simulink model "amon_model_full"  (R2025b)
settings: Solver=VariableStepAuto  StartTime=0.0  StopTime=1  RelTol=1e-3
values from neighbouring files (symbols this model uses):
  EDF_max = 100    [amon_model.m]
  EDF_min = 0    [amon_model.m]
  f_0_T = [0; 0; 0]    [amon_model.m]
  g = [0; 0; 9.81]    [amon_model.m]
  J = [0.02 0 0; 0 0.018 0; 0 0 0.03]    [amon_model.m]
  K_d = 0    [amon_model.m]
  k_fins = [1 1 1 1]    [amon_model.m]
  m = 2253    [amon_model.m]
  n_fins = [0  0  1 -1 ... (first row only)    [amon_model.m]
  r_fins = [   0.50  -0.50      0      0 ... (first row only)    [amon_model.m]
  r_T = [0; 0; 0]    [amon_model.m]
  servo1_offset = 0    [amon_model.m]
  servo2_offset = 0    [amon_model.m]
  servo3_offset = 0    [amon_model.m]
  servo4_offset = 0    [amon_model.m]
  servo_max = -45    [amon_model.m]
  servo_min = -45    [amon_model.m]
  tau_0_T = [0; 0; 0]    [amon_model.m]
  tau_edf = 0.2    [amon_model.m]
  tau_servo = 0.2    [amon_model.m]
libraries: aerolibconvert2 x4
settings Model: Creator=titit  LastModifiedBy=titit

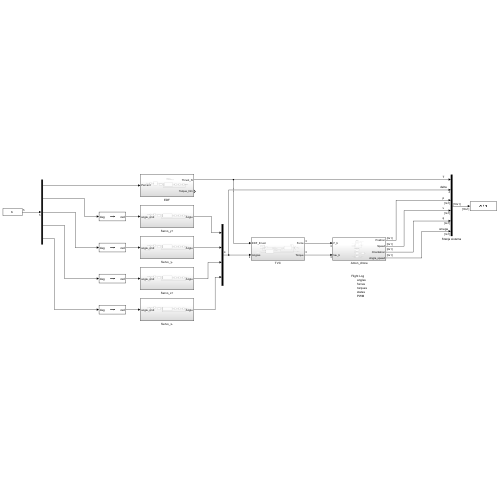
[thumbnail: Simulink's stored preview of the top-level diagram]
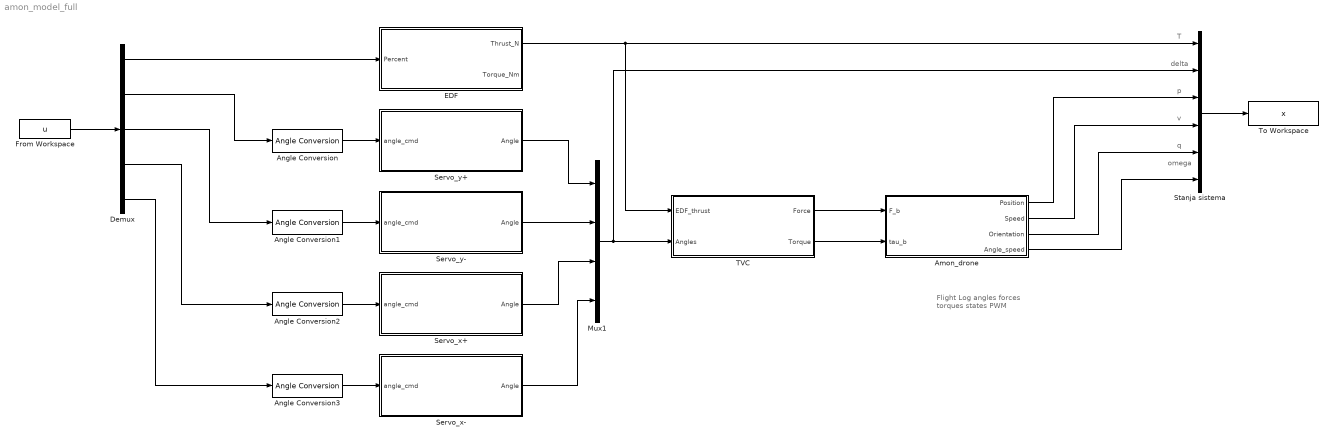
== system amon_model_full ==
  note: Flight Log
      | 	angles
      | 	forces
      | 	torques
      | 	states
      | 	PWM
  note: T
  note: delta
  note: p
  note: v
  note: q
  note: omega
  Amon_drone : Subsystem
  Angle Conversion{,1..3} (4 alike) : aerolibconvert2/Angle Conversion  IU=deg  OU=rad
  Demux : Demux  Outputs=5
  EDF : Subsystem
  From Workspace : FromWorkspace  VariableName=u
  Mux1 : Mux
  Servo_x+ : Subsystem
  Servo_x- : Subsystem
  Servo_y+ : Subsystem
  Servo_y- : Subsystem
  Stanja sistema : Mux  Inputs=6
  TVC : Subsystem
  To Workspace : ToWorkspace  VariableName=x  SaveFormat=Timeseries  SampleTime=-1
  wires:
  From Workspace/1 -> Demux/1
  Stanja sistema/1 -> To Workspace/1
  Demux/1 -> EDF/1(Percent)
  Demux/2 -> Angle Conversion/1
  Demux/3 -> Angle Conversion1/1
  Demux/4 -> Angle Conversion2/1
  Demux/5 -> Angle Conversion3/1
  Angle Conversion/1 -> Servo_y+/1(angle_cmd)
  Angle Conversion1/1 -> Servo_y-/1(angle_cmd)
  Angle Conversion2/1 -> Servo_x+/1(angle_cmd)
  Angle Conversion3/1 -> Servo_x-/1(angle_cmd)
  Servo_y+/1(Angle) -> Mux1/1
  Servo_y-/1(Angle) -> Mux1/2
  Servo_x+/1(Angle) -> Mux1/3
  Servo_x-/1(Angle) -> Mux1/4
  Mux1/1 -> Stanja sistema/2, TVC/2(Angles)
  EDF/1(Thrust_N) -> TVC/1(EDF_thrust), Stanja sistema/1
  TVC/1(Force) -> Amon_drone/1(F_b)
  TVC/2(Torque) -> Amon_drone/2(tau_b)
  Amon_drone/1(Position) -> Stanja sistema/3
  Amon_drone/2(Speed) -> Stanja sistema/4
  Amon_drone/3(Orientation) -> Stanja sistema/5
  Amon_drone/4(Angle_speed) -> Stanja sistema/6

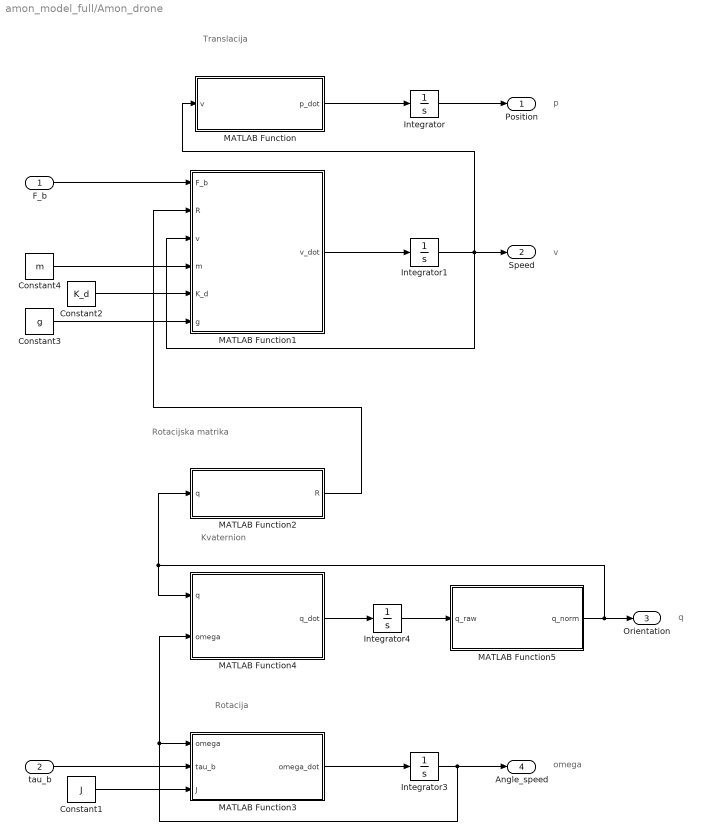
== system amon_model_full/Amon_drone ==
  note: p
  note: v
  note: q
  note: omega
  note: Translacija
  note: Kvaternion
  note: Rotacijska matrika
  note: Rotacija
  F_b : Inport
  tau_b : Inport  Port=2
  Constant1 : Constant  Value=J
  Constant2 : Constant  Value=K_d
  Constant3 : Constant  Value=g
  Constant4 : Constant  Value=m
  Integrator : Integrator
  Integrator1 : Integrator
  Integrator3 : Integrator  InitialCondition=[0;0;0]
  Integrator4 : Integrator
  MATLAB Function : MATLAB Function  TreatAsAtomicUnit=on
  MATLAB Function1 : MATLAB Function  TreatAsAtomicUnit=on
  MATLAB Function2 : MATLAB Function  TreatAsAtomicUnit=on
  MATLAB Function3 : MATLAB Function  TreatAsAtomicUnit=on
  MATLAB Function4 : MATLAB Function  TreatAsAtomicUnit=on
  MATLAB Function5 : MATLAB Function  TreatAsAtomicUnit=on
  Position : Outport
  Speed : Outport  Port=2
  Orientation : Outport  Port=3
  Angle_speed : Outport  Port=4
  wires:
  MATLAB Function/1(p_dot) -> Integrator/1
  Integrator/1 -> Position/1
  Integrator1/1 -> MATLAB Function/1(v), MATLAB Function1/3(v), Speed/1
  MATLAB Function1/1(v_dot) -> Integrator1/1
  MATLAB Function3/1(omega_dot) -> Integrator3/1
  Integrator3/1 -> MATLAB Function3/1(omega), MATLAB Function4/2(omega), Angle_speed/1
  F_b/1 -> MATLAB Function1/1(F_b)
  Constant4/1 -> MATLAB Function1/4(m)
  Constant2/1 -> MATLAB Function1/5(K_d)
  Constant3/1 -> MATLAB Function1/6(g)
  MATLAB Function2/1(R) -> MATLAB Function1/2(R)
  Constant1/1 -> MATLAB Function3/3(J)
  tau_b/1 -> MATLAB Function3/2(tau_b)
  MATLAB Function4/1(q_dot) -> Integrator4/1
  Integrator4/1 -> MATLAB Function5/1(q_raw)
  MATLAB Function5/1(q_norm) -> Orientation/1, MATLAB Function2/1(q), MATLAB Function4/1(q)

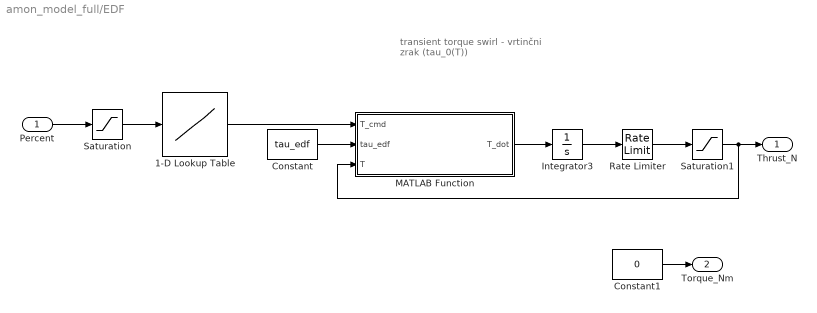
== system amon_model_full/EDF ==
  note: transient torque
      | swirl - vrtinčni zrak (tau_0(T))
  Percent : Inport
  1-D Lookup Table : Lookup_n-D  NumberOfTableDimensions=1  BreakpointsForDimension1=[-5:5]  Table=tanh([-5:5])  InternalRulePriority=Speed  RndMeth=Simplest
  Constant : Constant  Value=tau_edf
  Constant1 : Constant  Value=0
  Integrator3 : Integrator
  MATLAB Function : MATLAB Function  TreatAsAtomicUnit=on
  Rate Limiter : RateLimiter  SampleTimeMode=inherited
  Saturation : Saturate  UpperLimit=EDF_max  LowerLimit=EDF_min
  Saturation1 : Saturate  UpperLimit=100  LowerLimit=0
  Thrust_N : Outport
  Torque_Nm : Outport  Port=2
  wires:
  Percent/1 -> Saturation/1
  1-D Lookup Table/1 -> MATLAB Function/1(T_cmd)
  MATLAB Function/1(T_dot) -> Integrator3/1
  Saturation/1 -> 1-D Lookup Table/1
  Constant/1 -> MATLAB Function/2(tau_edf)
  Rate Limiter/1 -> Saturation1/1
  Saturation1/1 -> MATLAB Function/3(T), Thrust_N/1
  Constant1/1 -> Torque_Nm/1
  Integrator3/1 -> Rate Limiter/1

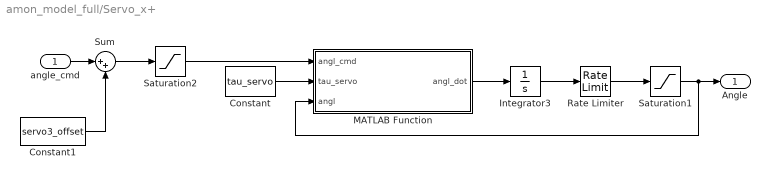
== system amon_model_full/Servo_x+ ==
  angle_cmd : Inport
  Constant : Constant  Value=tau_servo
  Constant1 : Constant  Value=servo3_offset
  Integrator3 : Integrator
  MATLAB Function : MATLAB Function  TreatAsAtomicUnit=on
  Rate Limiter : RateLimiter  SampleTimeMode=inherited
  Saturation1 : Saturate  UpperLimit=servo_max  LowerLimit=servo_min
  Saturation2 : Saturate  UpperLimit=servo_max  LowerLimit=servo_min
  Sum : Sum  Inputs=|++
  Angle : Outport
  wires:
  Sum/1 -> Saturation2/1
  Constant/1 -> MATLAB Function/2(tau_servo)
  MATLAB Function/1(angl_dot) -> Integrator3/1
  Saturation2/1 -> MATLAB Function/1(angl_cmd)
  Constant1/1 -> Sum/2
  angle_cmd/1 -> Sum/1
  Saturation1/1 -> MATLAB Function/3(angl), Angle/1
  Rate Limiter/1 -> Saturation1/1
  Integrator3/1 -> Rate Limiter/1

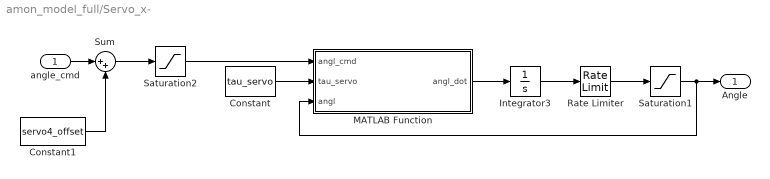
== system amon_model_full/Servo_x- ==
  angle_cmd : Inport
  Constant : Constant  Value=tau_servo
  Constant1 : Constant  Value=servo4_offset
  Integrator3 : Integrator
  MATLAB Function : MATLAB Function  TreatAsAtomicUnit=on
  Rate Limiter : RateLimiter  SampleTimeMode=inherited
  Saturation1 : Saturate  UpperLimit=servo_max  LowerLimit=servo_min
  Saturation2 : Saturate  UpperLimit=servo_max  LowerLimit=servo_min
  Sum : Sum  Inputs=|++
  Angle : Outport
  wires:
  Constant/1 -> MATLAB Function/2(tau_servo)
  MATLAB Function/1(angl_dot) -> Integrator3/1
  Saturation2/1 -> MATLAB Function/1(angl_cmd)
  Constant1/1 -> Sum/2
  angle_cmd/1 -> Sum/1
  Saturation1/1 -> MATLAB Function/3(angl), Angle/1
  Rate Limiter/1 -> Saturation1/1
  Sum/1 -> Saturation2/1
  Integrator3/1 -> Rate Limiter/1

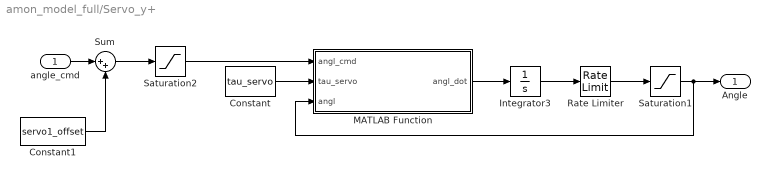
== system amon_model_full/Servo_y+ ==
  angle_cmd : Inport
  Constant : Constant  Value=tau_servo
  Constant1 : Constant  Value=servo1_offset
  Integrator3 : Integrator
  MATLAB Function : MATLAB Function  TreatAsAtomicUnit=on
  Rate Limiter : RateLimiter  SampleTimeMode=inherited
  Saturation1 : Saturate  UpperLimit=servo_max  LowerLimit=servo_min
  Saturation2 : Saturate  UpperLimit=servo_max  LowerLimit=servo_min
  Sum : Sum  Inputs=|++
  Angle : Outport
  wires:
  Saturation2/1 -> MATLAB Function/1(angl_cmd)
  MATLAB Function/1(angl_dot) -> Integrator3/1
  Saturation1/1 -> MATLAB Function/3(angl), Angle/1
  Constant/1 -> MATLAB Function/2(tau_servo)
  Rate Limiter/1 -> Saturation1/1
  angle_cmd/1 -> Sum/1
  Sum/1 -> Saturation2/1
  Constant1/1 -> Sum/2
  Integrator3/1 -> Rate Limiter/1

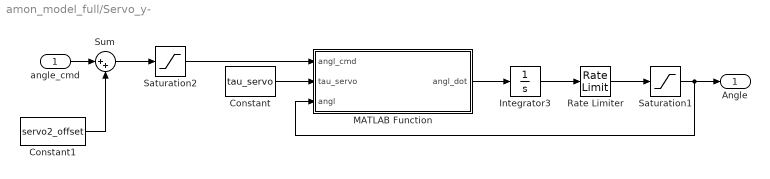
== system amon_model_full/Servo_y- ==
  angle_cmd : Inport
  Constant : Constant  Value=tau_servo
  Constant1 : Constant  Value=servo2_offset
  Integrator3 : Integrator
  MATLAB Function : MATLAB Function  TreatAsAtomicUnit=on
  Rate Limiter : RateLimiter  SampleTimeMode=inherited
  Saturation1 : Saturate  UpperLimit=servo_max  LowerLimit=servo_min
  Saturation2 : Saturate  UpperLimit=servo_max  LowerLimit=servo_min
  Sum : Sum  Inputs=|++
  Angle : Outport
  wires:
  Sum/1 -> Saturation2/1
  Constant/1 -> MATLAB Function/2(tau_servo)
  MATLAB Function/1(angl_dot) -> Integrator3/1
  Saturation2/1 -> MATLAB Function/1(angl_cmd)
  Constant1/1 -> Sum/2
  angle_cmd/1 -> Sum/1
  Saturation1/1 -> MATLAB Function/3(angl), Angle/1
  Rate Limiter/1 -> Saturation1/1
  Integrator3/1 -> Rate Limiter/1

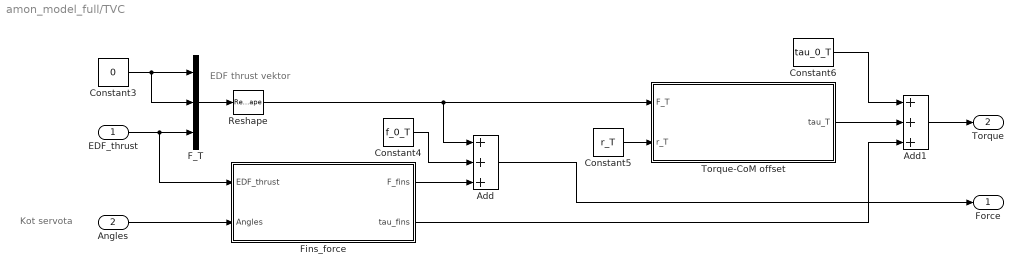
== system amon_model_full/TVC ==
  note: EDF thrust vektor
  note: Kot servota
  EDF_thrust : Inport
  Angles : Inport  Port=2
  Add : Sum  Inputs=+++
  Add1 : Sum  Inputs=+++
  Constant3 : Constant  Value=0
  Constant4 : Constant  Value=f_0_T
  Constant5 : Constant  Value=r_T
  Constant6 : Constant  Value=tau_0_T
  F_T : Mux  Inputs=3
  Fins_force : Subsystem
  Reshape : Reshape  OutputDimensionality=Column vector (2-D)
  Torque-CoM offset : Subsystem
  Force : Outport
  Torque : Outport  Port=2
  wires:
  EDF_thrust/1 -> Fins_force/1(EDF_thrust), F_T/3
  Constant3/1 -> F_T/2, F_T/1
  Angles/1 -> Fins_force/2(Angles)
  F_T/1 -> Reshape/1
  Constant5/1 -> Torque-CoM offset/2(r_T)
  Constant6/1 -> Add1/1
  Torque-CoM offset/1(tau_T) -> Add1/2
  Fins_force/2(tau_fins) -> Add1/3
  Add1/1 -> Torque/1
  Add/1 -> Force/1
  Fins_force/1(F_fins) -> Add/3
  Constant4/1 -> Add/2
  Reshape/1 -> Torque-CoM offset/1(F_T), Add/1

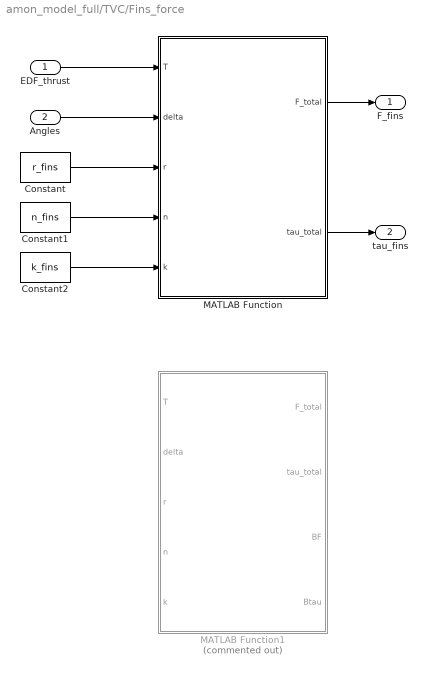
== system amon_model_full/TVC/Fins_force ==
  EDF_thrust : Inport
  Angles : Inport  Port=2
  Constant : Constant  Value=r_fins
  Constant1 : Constant  Value=n_fins
  Constant2 : Constant  Value=k_fins
  MATLAB Function : MATLAB Function  TreatAsAtomicUnit=on
  MATLAB Function1 : MATLAB Function  Commented=on  TreatAsAtomicUnit=on
  F_fins : Outport
  tau_fins : Outport  Port=2
  wires:
  EDF_thrust/1 -> MATLAB Function/1(T)
  MATLAB Function/1(F_total) -> F_fins/1
  Constant/1 -> MATLAB Function/3(r)
  Constant1/1 -> MATLAB Function/4(n)
  Constant2/1 -> MATLAB Function/5(k)
  MATLAB Function/2(tau_total) -> tau_fins/1
  Angles/1 -> MATLAB Function/2(delta)

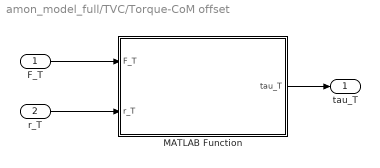
== system amon_model_full/TVC/Torque-CoM offset ==
  F_T : Inport
  r_T : Inport  Port=2
  MATLAB Function : MATLAB Function  TreatAsAtomicUnit=on
  tau_T : Outport
  wires:
  r_T/1 -> MATLAB Function/2(r_T)
  F_T/1 -> MATLAB Function/1(F_T)
  MATLAB Function/1(tau_T) -> tau_T/1

== matlab function amon_model_full/TVC/Torque-CoM offset/MATLAB Function ==
  data: F_T input; r_T input; tau_T output
function tau_T = tvc_block(F_T, r_T)
    tau_T = cross(r_T, F_T);
end

== matlab function amon_model_full/Amon_drone/MATLAB Function4 ==
  data: q input; omega input; q_dot output
function q_dot = quaternion_dynamics(q, omega)
    % Kvaternion / rotacijsko gibanje
    w_x = omega(1);
    w_y = omega(2);
    w_z = omega(3);

    Omega = [0,   -w_x, -w_y, -w_z;
             w_x,   0,   w_z, -w_y;
             w_y,  -w_z,  0,   w_x;
             w_z,   w_y, -w_x,  0];
    
    q_dot = (1/2) * Omega * q;

end

== matlab function amon_model_full/Amon_drone/MATLAB Function2 ==
  data: q input; R output
function R = q_to_R(q)
    qw = q(1);
    qx = q(2);
    qy = q(3);
    qz = q(4);
    
    % Rotacijska matrika
    R = [ 1 - 2*(qy^2 + qz^2), 2*(qx*qy - qw*qz),   2*(qx*qz + qw*qy);
          2*(qx*qy + qw*qz),   1 - 2*(qx^2 + qz^2), 2*(qy*qz - qw*qx);
          2*(qx*qz - qw*qy),   2*(qy*qz + qw*qx),   1 - 2*(qx^2 + qy^2)];
end

== matlab function amon_model_full/Amon_drone/MATLAB Function3 ==
  data: omega input; omega_dot output; tau_b input; J input
function omega_dot = rotational_dynamics(omega, tau_b, J)
    % Rotacijsko gibanje/Euler - tau_dist zanemarimo!
    % Matlab sintaksa: J^-1 = \
    omega_dot = J \ (tau_b - cross(omega, J * omega));
end

== matlab function amon_model_full/Amon_drone/MATLAB Function ==
  data: v input; p_dot output
function p_dot = position_kinematics(v)
    p_dot = v;
end

== matlab function amon_model_full/Amon_drone/MATLAB Function5 ==
  data: q_raw input; q_norm output
function q_norm = normalize_quaternion(q_raw)
    % Normalizacija
    n = norm(q_raw);
    
    if n < 1e-12
        q_norm = [1;0;0;0];
    else
        q_norm = q_raw / n;
    end

end

== matlab function amon_model_full/Servo_y+/MATLAB Function ==
  data: angl_cmd input; tau_servo input; angl_dot output; angl input
function angl_dot = servo_delay(angl_cmd, tau_servo, angl)
    angl_dot = (1/tau_servo) * (angl_cmd - angl);
end

== matlab function amon_model_full/EDF/MATLAB Function ==
  data: T_cmd input; tau_edf input; T_dot output; T input
function T_dot = thrust_delay(T_cmd, tau_edf, T)
    T_dot = (1/tau_edf) * (T_cmd - T);
end

== matlab function amon_model_full/Servo_y-/MATLAB Function ==
  data: angl_cmd input; tau_servo input; angl_dot output; angl input
function angl_dot = servo_delay(angl_cmd, tau_servo, angl)
    angl_dot = (1/tau_servo) * (angl_cmd - angl);
end

== matlab function amon_model_full/Servo_x+/MATLAB Function ==
  data: angl_cmd input; tau_servo input; angl_dot output; angl input
function angl_dot = servo_delay(angl_cmd, tau_servo, angl)
    angl_dot = (1/tau_servo) * (angl_cmd - angl);
end

== matlab function amon_model_full/Servo_x-/MATLAB Function ==
  data: angl_cmd input; tau_servo input; angl_dot output; angl input
function angl_dot = servo_delay(angl_cmd, tau_servo, angl)
    angl_dot = (1/tau_servo) * (angl_cmd - angl);
end

== matlab function amon_model_full/TVC/Fins_force/MATLAB Function1 ==
  data: T input; delta input; F_total output; r input; n input; k input; tau_total output; BF output; Btau output
function [F_total, tau_total, BF, Btau] = tvc_model_linear(T, delta, r, n, k)

    BF = zeros(3,4);
    Btau = zeros(3,4);
    
    for i = 1:4
        BF(:,i) = k(i) * n(:,i);
        Btau(:,i) = cross(r(:,i), BF(:,i));
    end
    
    delta = delta(:);
    %delta_eff = sin(delta(:));
    
    % skupna sila in momenti
    F_total = T * BF * delta;
    tau_total = T * Btau * delta;

end

== matlab function amon_model_full/TVC/Fins_force/MATLAB Function ==
  data: T input; delta input; F_total output; r input; n input; k input; tau_total output
function [F_total, tau_total] = tvc_model(T, delta, r, n, k)
    % delta_eff - mini aerodynamic model
    delta_eff = sin(delta);
    
    % sile posameznih finov
    %F_fins = T * n .* (k .* delta_eff');
    F_fins = zeros(3,4);

    for i = 1:4
        F_fins(:,i) = T * k(i) * delta_eff(i) * n(:,i);
    end
    
    % skupna sila
    F_total = sum(F_fins,2); % 2 - sum across the rows
    
    % momenti
    tau_total = sum(cross(r, F_fins, 1),2);
end

== matlab function amon_model_full/Amon_drone/MATLAB Function1 ==
  data: F_b input; R input; v input; v_dot output; m input; K_d input; g input
function v_dot = translational_dynamics(F_b, R, v, m, K_d, g)
    % Translacijsko gibanje
    v_dot = g + (1/m) * (R * F_b) - (1/m) * (K_d * v);
end
